simulink model "feedback_2D"  (R2022a)
settings: Solver=VariableStepAuto  StartTime=0.0  StopTime=1.0  MaxStep=1e-3  RelTol=1e-6
undefined symbols (not defined in the file): A_2D, B_2D, C_2D, K
settings Model: Creator=Orkun  LastModifiedBy=Orkun

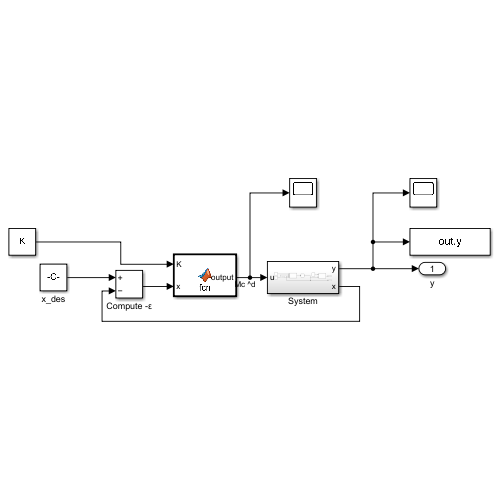
[thumbnail: Simulink's stored preview of the top-level diagram]
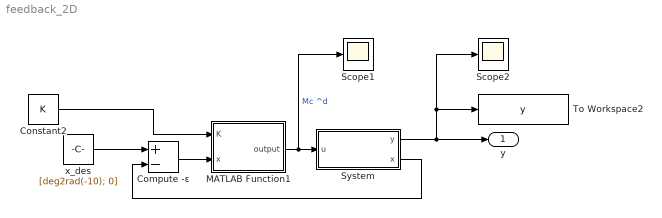
== system feedback_2D ==
  Compute -ε : Sum  Inputs=+-
  Constant2 : Constant  Value=K  VectorParams1D=off
  MATLAB Function1 : MATLAB Function  TreatAsAtomicUnit=on
  Scope1 : Scope
  Scope2 : Scope
  System : Subsystem
  To Workspace2 : ToWorkspace  VariableName=y  SaveFormat=Timeseries  SampleTime=-1
  x_des : Constant  Value=[deg2rad(-10); 0]
  y : Outport
  wires:
  System/1(y) -> y/1, Scope2/1, To Workspace2/1
  System/2(x) -> Compute -ε/2
  Constant2/1 -> MATLAB Function1/1(K)
  Compute -ε/1 -> MATLAB Function1/2(x)
  MATLAB Function1/1(output) -> Scope1/1, System/1(u)  "Mc ^d"
  x_des/1 -> Compute -ε/1

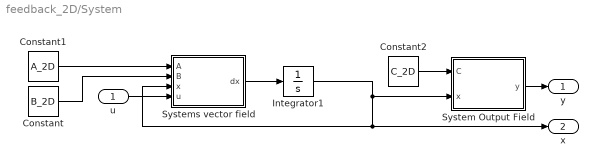
== system feedback_2D/System ==
  u : Inport
  Constant : Constant  Value=B_2D
  Constant1 : Constant  Value=A_2D
  Constant2 : Constant  Value=C_2D
  Integrator1 : Integrator  InitialCondition=[deg2rad(10);0]
  System Output Field : MATLAB Function  TreatAsAtomicUnit=on
  Systems vector field : MATLAB Function  TreatAsAtomicUnit=on
  y : Outport
  x : Outport  Port=2
  wires:
  Integrator1/1 -> x/1, Systems vector field/3(x), System Output Field/2(x)
  System Output Field/1(y) -> y/1
  Systems vector field/1(dx) -> Integrator1/1
  u/1 -> Systems vector field/4(u)
  Constant1/1 -> Systems vector field/1(A)
  Constant/1 -> Systems vector field/2(B)
  Constant2/1 -> System Output Field/1(C)

== matlab function feedback_2D/System/Systems vector field ==
  data: A input; B input; x input; u input; dx output
function dx = fcn(A, B, x, u)

%A = [0, 1, 0, 0; -11.8336, -0.5779, 358.5000, 1; 0, 0, -33.3333, 0; 0, 0, 0, 0];
%B = [0; 0; 33.3333; 0];


dx = (A*x) + (B*u);

== matlab function feedback_2D/System/System Output Field ==
  data: C input; x input; y output
function y = fcn(C, x)

%C = [1, 0, 0, 0; 0, 1, 0, 0];
y = C*x;

== matlab function feedback_2D/MATLAB Function1 ==
  data: K input; output output; x input
function output = fcn(K, x)

output = K*x;
